simulink library "vehicle_cl"  (R2018b)
settings: Solver=VariableStepAuto  StartTime=0.0  StopTime=10.0  RelTol=1e-3
undefined symbols (not defined in the file): initializeVariantsFromBlock, sim_param
libraries: modVehicle000_cl x1, vehicle000_cl x1, AyazOctLiftingBdy_cl x1, eulAng2RotMat_ul x1, thrAttachPtKinematics_ul x1, vehicleMMAdd x1
settings Model: Creator=mcobb  LastModifiedBy=jldanie5

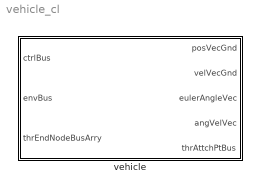
== system vehicle_cl ==
  vehicle : Subsystem  LoadFcn=initializeVariantsFromBlock(gcb)  InitFcn=initializeVariantsFromBlock(gcb)  StartFcn=initializeVariantsFromBlock(gcb)  Variant=on
      settings: PreSaveFcn=initializeVariantsFromBlock(gcb)

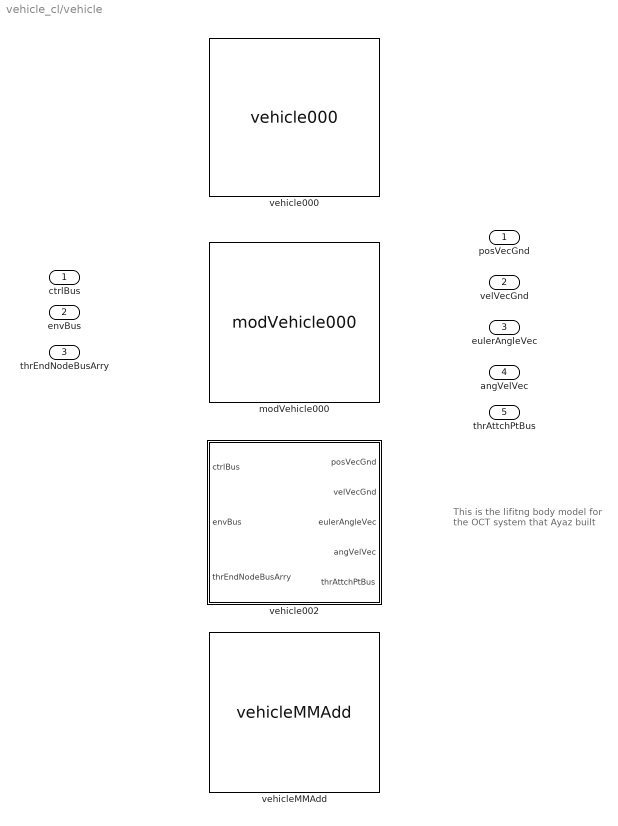
== system vehicle_cl/vehicle ==
  note: This is the lifitng body model for the OCT system that Ayaz built
  ctrlBus : Inport  OutDataTypeStr=Bus: ctrlBus
  envBus : Inport  Port=2  OutDataTypeStr=Bus: envBus
  thrEndNodeBusArry : Inport  Port=3
  modVehicle000 : modVehicle000_cl/modVehicle000  VariantControl=VSS_vehicle_modVehicle000  vcl=vhcl  rho=env.water.density.Value  grav=env.gravAccel.Value
  vehicle000 : vehicle000_cl/vehicle000  VariantControl=VSS_vehicle_vehicle000  vcl=vhcl  rho=env.water.density.Value  grav=env.gravAccel.Value
  vehicle002 : Subsystem  VariantControl=VSS_vehicle_vehicle002
      mask init:
      | load('OrginalOCctModelVars');
  vehicleMMAdd : vehicleMMAdd/vehicleMMAdd  VariantControl=VSS_vehicle_vehicleMMAdd  vcl=vhcl  rho=env.water.density.Value  grav=env.gravAccel.Value
  posVecGnd : Outport
  velVecGnd : Outport  Port=2
  eulerAngleVec : Outport  Port=3
  angVelVec : Outport  Port=4
  thrAttchPtBus : Outport  Port=5

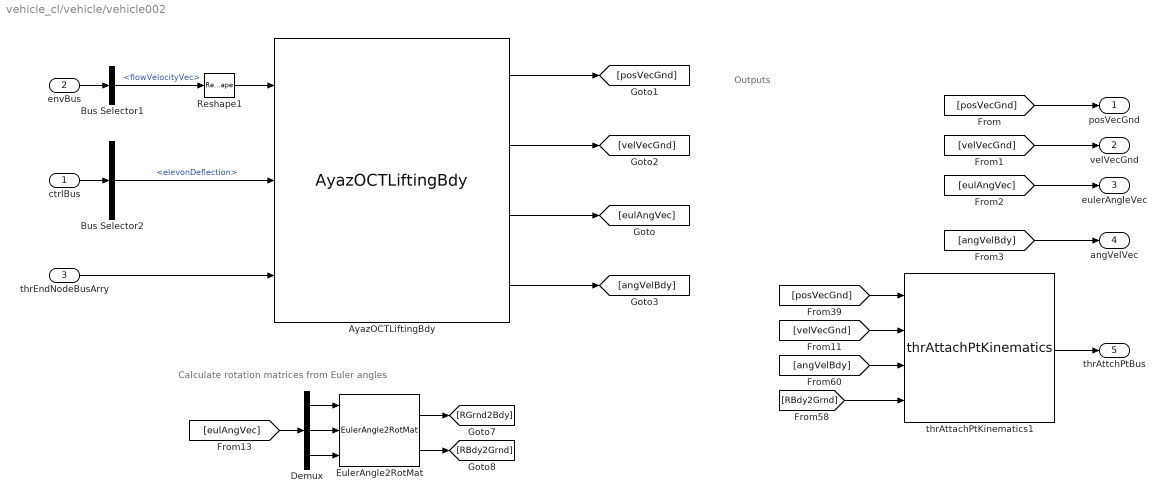
== system vehicle_cl/vehicle/vehicle002 ==
  note: Outputs
  note: Calculate rotation matrices from Euler angles
  ctrlBus : Inport  OutDataTypeStr=Bus: ctrlBus
  envBus : Inport  Port=2  OutDataTypeStr=Bus: envBus
  thrEndNodeBusArry : Inport  Port=3
  AyazOCTLiftingBdy : AyazOctLiftingBdy_cl/AyazOCTLiftingBdy  sim_param=sim_param  initCon=origOCT_iniCon
  Bus Selector1 : BusSelector  OutputSignals=flowVelocityVec
  Bus Selector2 : BusSelector  OutputSignals=elevonDeflection
  Demux : Demux  Outputs=3
  EulerAngle2RotMat : eulAng2RotMat_ul/EulerAngle2RotMat  SystemSampleTime=-1
  Reshape1 : Reshape  OutputDimensionality=Column vector (2-D)
  thrAttachPtKinematics1 : thrAttachPtKinematics_ul/thrAttachPtKinematics  atchPts=[sim_param.tether_imp_nodes.R1n_cm,sim_param.tether_imp_nodes.R2n_cm,sim_param.tether_imp_nodes.R3n_cm]
  posVecGnd : Outport
  velVecGnd : Outport  Port=2
  eulerAngleVec : Outport  Port=3
  angVelVec : Outport  Port=4
  thrAttchPtBus : Outport  Port=5
  wires:
  Bus Selector1/1 -> Reshape1/1  "<flowVelocityVec>"
  Reshape1/1 -> AyazOCTLiftingBdy/1
  envBus/1 -> Bus Selector1/1
  ctrlBus/1 -> Bus Selector2/1
  Bus Selector2/1 -> AyazOCTLiftingBdy/2  "<elevonDeflection>"
  thrEndNodeBusArry/1 -> AyazOCTLiftingBdy/3
  [posVecGnd] -> thrAttachPtKinematics1/1
  [RBdy2Grnd] -> thrAttachPtKinematics1/4
  thrAttachPtKinematics1/1 -> thrAttchPtBus/1
  [angVelBdy] -> thrAttachPtKinematics1/3
  [velVecGnd] -> thrAttachPtKinematics1/2
  Demux/3 -> EulerAngle2RotMat/3
  [eulAngVec] -> Demux/1
  Demux/2 -> EulerAngle2RotMat/2
  Demux/1 -> EulerAngle2RotMat/1
  EulerAngle2RotMat/1 -> [RGrnd2Bdy]
  EulerAngle2RotMat/2 -> [RBdy2Grnd]
  AyazOCTLiftingBdy/3 -> [eulAngVec]
  AyazOCTLiftingBdy/1 -> [posVecGnd]
  AyazOCTLiftingBdy/2 -> [velVecGnd]
  AyazOCTLiftingBdy/4 -> [angVelBdy]
  [posVecGnd] -> posVecGnd/1
  [velVecGnd] -> velVecGnd/1
  [eulAngVec] -> eulerAngleVec/1
  [angVelBdy] -> angVelVec/1
